simulink model "dawidek"  (R2013a)
settings: Solver=ode45  StartTime=0.0  StopTime=10  RelTol=1e-3
values from neighbouring files (symbols this model uses):
  A1 = 2    [cwiczenie8.m]    (also in cwiczenie8transmitancja.m; dawid.m)
  A2 = 4    [cwiczenie8.m]    (also in cwiczenie8transmitancja.m; dawid.m)
  Awe = 0.5    [dawid.m]
  Awy = 0.75    [dawid.m]
  czas_skoku = 2    [cwiczenie8.m]    (also in cwiczenie8transmitancja.m; dawid.m)
  du = 0.1*u0max    (= 0.3)    [cwiczenie8.m]    (also in cwiczenie8transmitancja.m; dawid.m)
  g = 10    [cwiczenie8.m]    (also in cwiczenie8transmitancja.m; dawid.m)
  h10 = u0/a1    [cwiczenie8.m]    (also in cwiczenie8transmitancja.m; dawid.m = u0*u0 / (Awy*Awy*2*g))
  h20 = u0/a2    [cwiczenie8.m]    (also in cwiczenie8transmitancja.m; dawid.m = u0*u0 / (Awe*Awe*2*g))
  u0 = tabu0(i)    [cwiczenie8.m]    (also in cwiczenie8transmitancja.m; dawid.m)
settings Model: Creator=LAB320-1552  LastModifiedBy=LAB320-1552

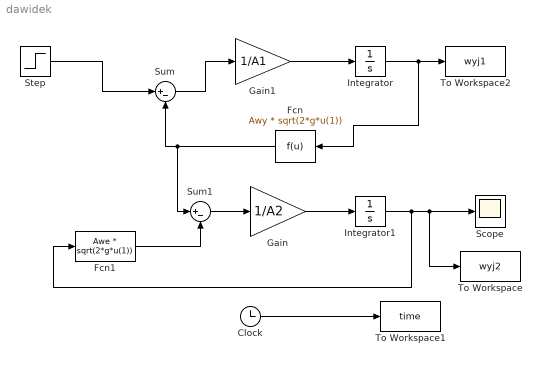
== system dawidek ==
  Clock : Clock
  Fcn : Fcn  Expr=Awy * sqrt(2*g*u(1))
  Fcn1 : Fcn  Expr=Awe * sqrt(2*g*u(1))
  Gain : Gain  Gain=1/A2
  Gain1 : Gain  Gain=1/A1
  Integrator : Integrator  InitialCondition=h10
  Integrator1 : Integrator  InitialCondition=h20
  Scope : Scope
  Step : Step  Time=czas_skoku  Before=u0  After=u0+du  SampleTime=0
  Sum : Sum  Inputs=|+-
  Sum1 : Sum  Inputs=|+-
  To Workspace : ToWorkspace  VariableName=wyj2  SampleTime=-1
  To Workspace1 : ToWorkspace  VariableName=time  SampleTime=-1
  To Workspace2 : ToWorkspace  VariableName=wyj1  SampleTime=-1
  wires:
  Step/1 -> Sum/1
  Sum/1 -> Gain1/1
  Gain1/1 -> Integrator/1
  Fcn1/1 -> Sum1/2
  Sum1/1 -> Gain/1
  Gain/1 -> Integrator1/1
  Integrator1/1 -> Fcn1/1, To Workspace/1, Scope/1
  Clock/1 -> To Workspace1/1
  Integrator/1 -> Fcn/1, To Workspace2/1
  Fcn/1 -> Sum/2, Sum1/1
